simulink model "PBMRAC_Baseline_Model"  (R2024a)
settings: Solver=VariableStepAuto  StartTime=0.0  StopTime=10.0  RelTol=1e-3
undefined symbols (not defined in the file): a_e_tilde, K_p, K_v, Lambda_tilde, p_i_0, v_i_0
settings Model: Creator=Usuario  LastModifiedBy=Usuario

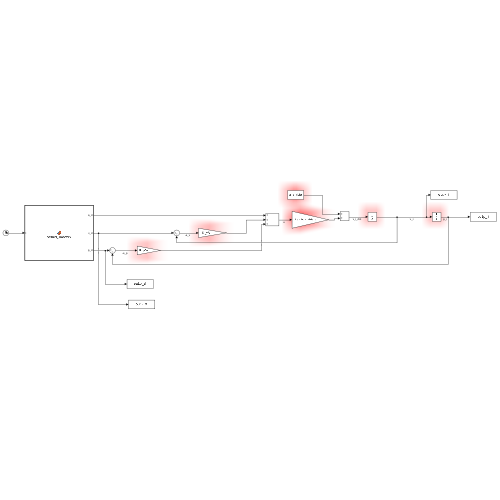
[thumbnail: Simulink's stored preview of the top-level diagram]
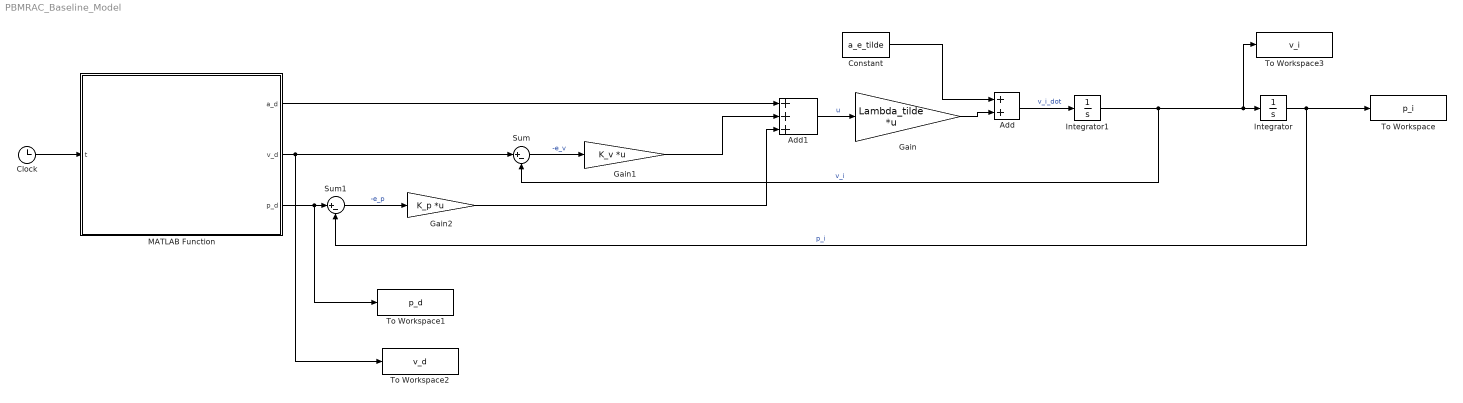
== system PBMRAC_Baseline_Model ==
  Add : Sum
  Add1 : Sum  Inputs=+++
  Clock : Clock
  Constant : Constant  Value=a_e_tilde
  Gain : Gain  Gain=Lambda_tilde  Multiplication=Matrix(K*u)
  Gain1 : Gain  Gain=K_v  Multiplication=Matrix(K*u)
  Gain2 : Gain  Gain=K_p  Multiplication=Matrix(K*u)
  Integrator : Integrator  InitialCondition=p_i_0
  Integrator1 : Integrator  InitialCondition=v_i_0
  MATLAB Function : MATLAB Function  TreatAsAtomicUnit=on
  Sum : Sum  Inputs=|+-
  Sum1 : Sum  Inputs=|+-
  To Workspace : ToWorkspace  VariableName=p_i  SaveFormat=Timeseries  SampleTime=-1
  To Workspace1 : ToWorkspace  VariableName=p_d  SaveFormat=Timeseries  SampleTime=-1
  To Workspace2 : ToWorkspace  VariableName=v_d  SaveFormat=Timeseries  SampleTime=-1
  To Workspace3 : ToWorkspace  VariableName=v_i  SaveFormat=Timeseries  SampleTime=-1
  wires:
  Add/1 -> Integrator1/1  "v_i_dot"
  Integrator1/1 -> Sum/2, To Workspace3/1, Integrator/1  "v_i"
  Integrator/1 -> Sum1/2, To Workspace/1  "p_i"
  Clock/1 -> MATLAB Function/1(t)
  Constant/1 -> Add/1
  Gain/1 -> Add/2
  Add1/1 -> Gain/1  "u"
  MATLAB Function/1(a_d) -> Add1/1
  MATLAB Function/2(v_d) -> To Workspace2/1, Sum/1
  MATLAB Function/3(p_d) -> To Workspace1/1, Sum1/1
  Sum/1 -> Gain1/1  "-e_v"
  Sum1/1 -> Gain2/1  "-e_p"
  Gain1/1 -> Add1/2
  Gain2/1 -> Add1/3

== matlab function PBMRAC_Baseline_Model/MATLAB Function ==
  data: a_d output; v_d output; t input; p_d output; dir parameter
function [a_d,v_d,p_d]=desired_trajectory(t,dir)
p_d=dir;
v_d=[0;0;0];
a_d=[0;0;0];
end
